simulink library "carnot"  (R2013b)
settings: Solver=ode45  StartTime=0.0  StopTime=10.0  RelTol=1e-3
undefined symbols (not defined in the file or in its folder): A, acol, Ahabit, Awin, Azimuth_Angle, AziWin, B, C, c1, c4, capc, caph, CarnotCallbacks_Density, CarnotCallbacks_Enthalpy, CarnotCallbacks_Enthalpy2Temperature, CarnotCallbacks_Entropy, CarnotCallbacks_Evaporation_Enthalpy, CarnotCallbacks_GlobalMessageLevel, CarnotCallbacks_Grashof, CarnotCallbacks_Heat_Capacity, CarnotCallbacks_Kinematic_Viscosity, CarnotCallbacks_Prandtl, CarnotCallbacks_Saturation_Property, CarnotCallbacks_Saturation_Temperature, CarnotCallbacks_Saturation_Value_Water, CarnotCallbacks_Specific_Volume, CarnotCallbacks_Thermal_Conductivity, CarnotCallbacks_Vapour_Content, CarnotCallbacks_Vapour_Pressure, con, cond, d, Dd, density, dfin, dia, DiameterLastPiece, DPConstant, dpipe, DPLinear, DPQuadratic, emission_out, fluid, FluidMix, FluidType, FPC, frame, g, GeodeticHeight, Gwin, heat_capacity, hgt, HP, Hroom, ID, inlet, K, l, lin, lpipe ... (+29)
undefined symbols (not defined in the file): c2, c3, c5, c6, cwall, dactive, height, mc, mID, rho, tau, UAneighbour, UAwall, uloss
libraries: carnot x333, simulink x25, simulink_extras x7
(part 16 of 16)

== system carnot/Storage/Thermal/Storage_Ports/Pipe_stratified/T_criteria not satisfied ==
  Action Port : ActionPort
  MATLAB Fcn1 : MATLABFcn  MATLABFcn=[zeros(u-1,1); 1; zeros(nodes-u,1)]  OutputDimensions=nodes
  const : Constant  Value=outlet
  Out1 : Outport  OutputWhenDisabled=reset  InitialOutput=0
  wires:
  const/1 -> MATLAB Fcn1/1
  MATLAB Fcn1/1 -> Out1/1

== system carnot/Storage/Thermal/Storage_Ports/Pipe_stratified/massflow downwards ==
  In1 : Inport
  Action Port : ActionPort
  MATLAB Fcn : MATLABFcn  MATLABFcn=find(u,1,'last')+outlet-1  OutputDimensions=1
  MATLAB Fcn1 : MATLABFcn  MATLABFcn=[zeros(u-1,1); 1; zeros(nodes-u,1)]  OutputDimensions=nodes
  Out1 : Outport
  wires:
  MATLAB Fcn/1 -> MATLAB Fcn1/1
  In1/1 -> MATLAB Fcn/1
  MATLAB Fcn1/1 -> Out1/1

== system carnot/Storage/Thermal/Storage_Ports/Pipe_stratified/massflow upwards ==
  In1 : Inport
  Action Port : ActionPort
  MATLAB Fcn : MATLABFcn  MATLABFcn=find(u,1,'first')+inlet-1  OutputDimensions=1
  MATLAB Fcn1 : MATLABFcn  MATLABFcn=[zeros(u-1,1); 1; zeros(nodes-u,1)]  OutputDimensions=nodes
  Out1 : Outport
  wires:
  In1/1 -> MATLAB Fcn/1
  MATLAB Fcn/1 -> MATLAB Fcn1/1
  MATLAB Fcn1/1 -> Out1/1

== system carnot/Storage/Thermal/surface_models/Open_Surface/add 5.6 ==
  In1 : Inport
  Sum : Sum  SaturateOnIntegerOverflow=on  InputSameDT=on  OutDataTypeStr=Inherit: Same as first input
  const : Constant  Value=c
  Out1 : Outport
  wires:
  const/1 -> Sum/1
  In1/1 -> Sum/2
  Sum/1 -> Out1/1

== system carnot/Load/Houses/heat_transfer/alfa_window_in/transmission coefficient 1-2-3-4-layer(s)/LUT_taualfa ==
  note: NOTE: The TAUALFA-Lookup-table is calculated with "taualfa.m"
      | for 4 mm glass, but you can use it also for  3, 4, 6 or 8 mm glass.
      | The mistake is neglectable (see results in "taulut.m").
  note: transmission coefficient TAUALFA of a window glass with 1,2,3 or 4 layers
  note: (from: Duffie / Beckman: Solar Engineering of Thermal Processes, 1991
  teta : Inport
  numlayer : Inport  Port=2
  "TAUALFA 1-2-3-4 layers, standardized to 1.0, (4 mm float glass, no dirt absorption, 97% room absorption)" : Lookup2D  RowIndex=[0:10:90]  ColumnIndex=[1:4]  Table=[1.0000 1.0000 1.0000 1.0000; 0.9996 0.9991 0.9987 0.9983; 0.9979 0.9961 0.9945 0.9929; 0.9937 0.9894 0.9861 0.9836; 0.9839 0.9753 0.9704 0.9680; 0.9608 0.9438 0.9365 0.9361; 0.9061 0.8679 0.8484 0.8413; 0.7755 0.6821 0.6182 0.5717; 0.4807 0.3277 0.2324 0.1688; 0 0 0 0]  SaturateOnIntegerOverflow=on  InputSameDT=on
  tau : Outport
  wires:
  teta/1 -> "TAUALFA 1-2-3-4 layers, standardized to 1.0, (4 mm float glass, no dirt absorption, 97% room absorption)"/1
  numlayer/1 -> "TAUALFA 1-2-3-4 layers, standardized to 1.0, (4 mm float glass, no dirt absorption, 97% room absorption)"/2
  "TAUALFA 1-2-3-4 layers, standardized to 1.0, (4 mm float glass, no dirt absorption, 97% room absorption)"/1 -> tau/1

== system carnot/Load/Houses/room_nodes/Room_Node/convective_node/Mean ==
  u1 : Inport
  u2 : Inport  Port=2
  Sum : Sum  SaturateOnIntegerOverflow=on  InputSameDT=on  OutDataTypeStr=Inherit: Same as first input
  gain : Gain  Gain=0.5  SaturateOnIntegerOverflow=on  OutDataTypeStr=Inherit: Same as input  ParamDataTypeStr=Inherit: Same as input
  Mean : Outport
  wires:
  Sum/1 -> gain/1
  u1/1 -> Sum/1
  gain/1 -> Mean/1
  u2/1 -> Sum/2

== system carnot/Load/Houses/room_nodes/Room_Node/convective_node/Subsystem ==
  note: (J/(kg*K)
  T : Inport
  Celsius2Kelvin : Bias  Bias=273.15
  air_gas_constant : Gain  Gain=287  SaturateOnIntegerOverflow=on  OutDataTypeStr=Inherit: Same as input  ParamDataTypeStr=Inherit: Same as input
  R*T ' : Outport
  wires:
  air_gas_constant/1 -> R*T '/1
  T/1 -> Celsius2Kelvin/1
  Celsius2Kelvin/1 -> air_gas_constant/1

== system carnot/Load/Houses/wall_floor/Window_with_Shading/alfa_window_in/transmission_absorption ==
  note: 1. solar radiation into room (behind window glass layers)
      | 2. absorbed solar radiation flowing from inner window surface into zone
  note: Assumption:
      | 1. gvalue = gvalue(0)
      | 2. gvalue(teta) / gvalue = tau(teta) / tau(0)
  sun_t : Inport
  WDB : Inport  Port=2
  control : Inport  Port=3
  Demux : Demux  Outputs=2
  Demux1 : Demux  Outputs=3
  LUT_taualfa : Subsystem  mask(LOOK UP TABLE){}
      mask help:
      | Normalized RADIATION TRANSMISSION COEFFICIENT of a window glass layer stack with 1, 2, 3 or 4 layers depending on the incidence angle.
      |
      | teta		: incidence angle = angle between surface normal and
      | 	                incidence direction, degree
      | numlayer	: number of layers within the window glass, [1,4].
      | tau		: transmission of glass layer stack, [0,1]
      |
      | NOTE: This block is defined for pane thickness between 3 and 6 mm.
  Mux : Mux  Inputs=2
  Product{1..4,7..8} (6 alike) : Product  SaturateOnIntegerOverflow=on  RndMeth=Zero  InputSameDT=on  OutDataTypeStr=Inherit: Same as first input
  Product11 : Product  Inputs=**  SaturateOnIntegerOverflow=on  RndMeth=Zero  InputSameDT=on  OutDataTypeStr=Inherit: Same as first input
  Shading : Subsystem
  Sum : Sum  Inputs=+-  SaturateOnIntegerOverflow=on  InputSameDT=on  OutDataTypeStr=Inherit: Same as first input
  Sum3 : Sum  SaturateOnIntegerOverflow=on  InputSameDT=on  OutDataTypeStr=Inherit: Same as first input
  const1 : Constant  Value=gvalue
  numlayer : Constant  Value=numpanes
  tau(0) : Gain  Gain=tauzero  SaturateOnIntegerOverflow=on  OutDataTypeStr=Inherit: Same as input  ParamDataTypeStr=Inherit: Same as input
  teta(taudfu) : Constant  Value=60
  qdot_abs : Outport
  qdot_sol : Outport  Port=2
  wires:
  Mux/1 -> LUT_taualfa/2(teta)
  numlayer/1 -> LUT_taualfa/1(numlpanes)
  teta(taudfu)/1 -> Mux/2
  Demux1/1 -> Mux/1  "teta"
  Sum/1 -> qdot_abs/1
  Product11/1 -> Sum/1  "qdot_room"
  Demux/2 -> Product8/1  "tau_norm(60)"
  Sum3/1 -> tau(0)/1, Product11/2
  Product8/1 -> Sum3/2
  Product7/1 -> Sum3/1
  Demux/1 -> Product7/1  "tau_norm(teta)"
  LUT_taualfa/1(tau_norm) -> Demux/1  "Qdot_sol"
  sun_t/1 -> Demux1/1
  tau(0)/1 -> Product3/1
  Product3/1 -> Sum/2, qdot_sol/1
  Demux1/3 -> Product1/1  "Idfu_t"
  Product1/1 -> Product8/2
  Demux1/2 -> Product2/1  "Idir_t"
  Product2/1 -> Product7/2
  Shading/1(f_dir) -> Product2/2
  Shading/2(f_dfu) -> Product1/2
  Shading/4(f_tau) -> Product3/2
  Product4/1 -> Product11/1
  const1/1 -> Product4/1
  Shading/3(f_g) -> Product4/2
  WDB/1 -> Shading/1(WDB)
  control/1 -> Shading/2(control)

== system carnot/Source/Chiller/Cooling_Tower/Verbrauch // consumption/Verdunstung/Enthalpie  ==
  x_le : Inport
  t_le : Inport  Port=2
  Add : Sum
  Add1 : Sum
  Product : Product  RndMeth=Zero
  Product1 : Product  RndMeth=Zero
  Product2 : Product  RndMeth=Zero
  cp_d : Constant  Value=1.861
  cp_lt : Constant  Value=1.006
  dhv0 : Constant  Value=2500
  h_le : Outport
  wires:
  Add/1 -> h_le/1
  cp_lt/1 -> Product/1
  t_le/1 -> Product/2, Product2/1
  Product/1 -> Add/1
  Product1/1 -> Add/2
  x_le/1 -> Product1/1
  cp_d/1 -> Product2/2
  Add1/1 -> Product1/2
  Product2/1 -> Add1/1
  dhv0/1 -> Add1/2

== system carnot/Load/Houses/wall_floor/Window_with_Shading/alfa_window_in/transmission_absorption/LUT_taualfa ==
  note: Normalized radiation transmission TAUALFA
      | of a window glass stack with 1,2,3 or 4 layers
  note: NOTE:
      | TAUALFA-Lookup-table calculated with "taualfa.m":
      |   a) 4mm float glass (error neglectable if glass thickness is 3 or 6mm),
      |   b) no dirt absorption on glass surfaces,
      |   c) 100% room absorption,
      |   d) normalized to tau(0).
      |
      | From: Duffie / Beckman: Solar Engineering of Thermal Processes, 1991
  numlpanes : Inport
  teta : Inport  Port=2
  TAUALFA 1-2-3-4 layers : Lookup2D  RowIndex=[0:10:90]  ColumnIndex=[1:4]  Table="[1  1  1  1;.99955 .99912  .9987 .99827;.99787  .9961 .99449 .99298;.99364 .98941 .98618 .98366;.98364 .97519 .97041 .96824;.9601 .94337 .93638 .93624;.90423 .86634 .84734 .84064;.77129 .67843 .61507 .56891;.47436  .3235 .22952 .16682;0  0  0  0]"  SaturateOnIntegerOverflow=on  InputSameDT=on
  tau_norm : Outport
  wires:
  TAUALFA 1-2-3-4 layers/1 -> tau_norm/1
  numlpanes/1 -> TAUALFA 1-2-3-4 layers/2
  teta/1 -> TAUALFA 1-2-3-4 layers/1

== system carnot/Load/Houses/wall_floor/Window_with_Shading/alfa_window_in/transmission_absorption/Shading ==
  WDB : Inport
  control : Inport  Port=2
  Bus Selector : BusSelector  OutputSignals=Zenith_Angle
  Demux : Demux
  Mux : Mux  Inputs=2
  S-Function : S-Function  FunctionName=venetian  Parameters=bli_a, bli_b, bli_c, bli_d, bli_alpha, bli_refl, shad_type, type_glazing, tau_shad  EnableBusSupport=off
  f_dir : Outport
  f_dfu : Outport  Port=2
  f_g : Outport  Port=3
  f_tau : Outport  Port=4
  wires:
  Demux/4 -> f_tau/1
  Demux/3 -> f_g/1
  Demux/2 -> f_dfu/1
  Demux/1 -> f_dir/1
  S-Function/1 -> Demux/1
  Mux/1 -> S-Function/1
  control/1 -> Mux/1
  Bus Selector/1 -> Mux/2  "<Zenith_Angle>"
  WDB/1 -> Bus Selector/1

== matlab function carnot/Source/Chiller/Cooling_Tower/Leistungseinflüsse // influence on coolingpower/t_ia_ist /isnan ==
  data: u input; y output

function y = fcn(u)

%Verhindert die Fehlerausgabe bei Teilen durch den Wert 0 
%Dieser Zustand tritt ein wenn der Volumenstrom 0 l/s gesetzt wird.

v = isnan (u);

if v == 0
    
    y = u;

else 
    
    y = 0;
    
end

== matlab function carnot/Source/Chiller/Compression_Air_Water_Chiller/cooling/isinf ==
  data: u input; y output

function y = fcn(u)

% Avoids errors when dividing by very small values. 
% This situation appears when the massflow is near zero.

v = isinf (u);

if v == 0
    
    y = u;

else 
    
    y = 0;
    
end

== matlab function carnot/Source/Chiller/Compression_Air_Water_Chiller/cooling/isnan ==
  data: u input; y output

function y = fcn(u)

% Avoids errors when dividing by zero. 
% This situation appears when the massflow is zero.

v = isnan (u);

if v == 0
    
    y = u;

else 
    
    y = 0;
    
end
